simulink model "IEEE123bus_v2019b_Phasor_PI"  (R2019b)
settings: Solver=ode4  StartTime=0.0  StopTime=100  FixedStep=Ts  MaxStep=1e-4  RelTol=1e-3
InitFcn:
  | a=1; % Loading Factor
  | Ts=0.1;% For Delay Blocks in Voltage Regulator Controls
  | % phase to sequence conversion of RXB matrices
  | c=1*exp(sqrt(-1)*(120*pi/180));
  | T=[1 1 1;1 c*c c;1 c c*c];
  | Tinv=1/3*[1 1 1;1 c c*c;1 c*c c];
  | 
  | % Simulation data for the IEEE 123 Node Test Feeder model
  | mi2km = 1.60934;%  miles to km conversion
  | ft2km = 0.0003048; % feet to km conversion
  | ms2F = 1*1e-6/(2*pi*60);% microsiemens to Farads conversion
  | 
  | %% Configuration 1
  | % Series Resitance and Reactance - ohm/mile
  | R_1 = [0.4576 0.1560 0.1535;0.1560 0.4666 0.1580;0.1535 0.1580 0.4615];
  | X_1 = [1.0780 0.5017 0.3849;0.5017 1.0482 0.4236;0.3849 0.4236 1.0651];
  | % charging susceptance - microsiemens/mile
  | B_1 = [5.6765 -1.8319 -0.6982;-1.8319 5.9809 -1.1645;-0.6982 -1.1645 5.3971];
  | 
  | R_1 = R_1/mi2km;
  | Rseq=Tinv*R_1*T;
  | R1_1=Rseq(2,2);R0_1=Rseq(1,1);
  | 
  | L_1 = (X_1/(2*pi*60))/mi2km;
  | Lseq=Tinv*L_1*T;
  | L1_1=Lseq(2,2);L0_1=Lseq(1,1);
  | 
  | C_1 =(B_1*ms2F)/mi2km;
  | Cseq=Tinv*C_1*T;
  | C1_1=Cseq(2,2);C0_1=Cseq(1,1);
  | %% Configuration 2 - series reactance - ohm/mile
  | R_2 = [0.4666 0.1580 0.1560;0.1580 0.4615 0.1535;0.1560 0.1535 0.4576];
  | X_2 = [1.0482 0.4236 0.5017;0.4236 1.0651 0.3849;0.5017 0.3849 1.0780];
  | % charging susceptance - microsiemens/mile
  | B_2 = [5.9809 -1.1645 -1.8319;-1.1645 5.3971 -0.6982;-1.8319 -0.6982 5.6765];
  | 
  | R_2 = R_2/mi2km;
  | Rseq=Tinv*R_2*T;
  | R1_2=Rseq(2,2);R0_2=Rseq(1,1);
  | 
  | L_2 = (X_2/(2*pi*60))/mi2km;
  | Lseq=Tinv*L_2*T;
  | L1_2=Lseq(2,2);L0_2=Lseq(1,1);
  | 
  | C_2 =(B_2*ms2F)/mi2km;
  | Cseq=Tinv*C_2*T;
  | C1_2=Cseq(2,2);C0_2=Cseq(1,1);
  | %% Configuration 3 - series reactance - ohm/mile
  | R_3 = [0.4615 0.1535 0.1580;0.1535 0.4576 0.1560;0.1580 0.1560 0.4666];
  | X_3 = [1.0651 0.3849 0.4236;0.3849 1.0780 0.5017;0.4236 0.5017 1.0482];
  | % charging susceptance - microsiemens/mile
  | B_3 = [5.3971 -0.6982 -1.1645;-0.6982 5.6765 -1.8319; -1.1645 -1.8319 5.9809];
  | 
  | R_3 = R_3/mi2km;
  | Rseq=Tinv*R_3*T;
  | R1_3=Rseq(2,2);R0_3=Rseq(1,1);
  | 
  | L_3 = (X_3/(2*pi*60))/mi2km;
  | Lseq=Tinv*L_3*T;
  | L1_3=Lseq(2,2);L0_3=Lseq(1,1);
  | ... (+157 lines)
undefined symbols (not defined in the file or in its folder): D1, Delta, find_system, j
libraries: powerlib x771, powerlib_meascontrol x31
(part 3 of 7)

== system IEEE123bus_v2019b_Phasor_PI/38 ==
  2 : powerlib/Measurements/Three-Phase V-I Measurement  VoltageMeasurement=phase-to-ground  SetLabelV=on  LabelV=V38  Vpu=off  VpuLL=off  CurrentMeasurement=no  SetLabelI=on  LabelI=I800  Ipu=off  Pbase=100e6  Vbase=24900  OutputType=Complex  PhasorSimulation=on  PSBequivalent=0
      settings: SourceProductName=Simscape Electrical
  Ground82 : powerlib/Elements/Ground  LConnTagsString=a
      settings: SourceProductName=Simscape Electrical
  Ground83 : powerlib/Elements/Ground  LConnTagsString=a
      settings: SourceProductName=Simscape Electrical
  b : PMIOPort  Side=Right
  B : PMIOPort  Port=2  Side=Left
  connections:
  Ground82/LConn1 -- 2/RConn3 -- 2/RConn1
  Ground83/LConn1 -- 2/LConn3 -- 2/LConn1
  2/RConn2 -- b/RConn1
  2/LConn2 -- B/RConn1

== system IEEE123bus_v2019b_Phasor_PI/39 ==
  2 : powerlib/Measurements/Three-Phase V-I Measurement  VoltageMeasurement=phase-to-ground  SetLabelV=on  LabelV=V39  Vpu=off  VpuLL=off  CurrentMeasurement=no  SetLabelI=on  LabelI=I800  Ipu=off  Pbase=100e6  Vbase=24900  OutputType=Complex  PhasorSimulation=on  PSBequivalent=0
      settings: SourceProductName=Simscape Electrical
  Ground82 : powerlib/Elements/Ground  LConnTagsString=a
      settings: SourceProductName=Simscape Electrical
  Ground83 : powerlib/Elements/Ground  LConnTagsString=a
      settings: SourceProductName=Simscape Electrical
  b : PMIOPort  Side=Right
  B : PMIOPort  Port=2  Side=Left
  connections:
  2/LConn2 -- B/RConn1
  2/RConn2 -- b/RConn1
  2/LConn1 -- 2/LConn3 -- Ground83/LConn1
  2/RConn1 -- 2/RConn3 -- Ground82/LConn1

== system IEEE123bus_v2019b_Phasor_PI/4 ==
  2 : powerlib/Measurements/Three-Phase V-I Measurement  VoltageMeasurement=phase-to-ground  SetLabelV=on  LabelV=V4  Vpu=off  VpuLL=off  CurrentMeasurement=no  SetLabelI=on  LabelI=I4  Ipu=off  Pbase=100e6  Vbase=24900  OutputType=Complex  PhasorSimulation=on  PSBequivalent=0
      settings: SourceProductName=Simscape Electrical
  Ground82 : powerlib/Elements/Ground  LConnTagsString=a
      settings: SourceProductName=Simscape Electrical
  Ground83 : powerlib/Elements/Ground  LConnTagsString=a
      settings: SourceProductName=Simscape Electrical
  c : PMIOPort  Side=Right
  C : PMIOPort  Port=2  Side=Left
  connections:
  Ground83/LConn1 -- 2/LConn1 -- 2/LConn2
  Ground82/LConn1 -- 2/RConn1 -- 2/RConn2
  c/RConn1 -- 2/RConn3
  C/RConn1 -- 2/LConn3

== system IEEE123bus_v2019b_Phasor_PI/41 ==
  2 : powerlib/Measurements/Three-Phase V-I Measurement  VoltageMeasurement=phase-to-ground  SetLabelV=on  LabelV=V41  Vpu=off  VpuLL=off  CurrentMeasurement=no  SetLabelI=on  LabelI=I800  Ipu=off  Pbase=100e6  Vbase=24900  OutputType=Complex  PhasorSimulation=on  PSBequivalent=0
      settings: SourceProductName=Simscape Electrical
  Ground82 : powerlib/Elements/Ground  LConnTagsString=a
      settings: SourceProductName=Simscape Electrical
  Ground83 : powerlib/Elements/Ground  LConnTagsString=a
      settings: SourceProductName=Simscape Electrical
  c : PMIOPort  Side=Right
  C : PMIOPort  Port=2  Side=Left
  connections:
  2/LConn1 -- 2/LConn2 -- Ground83/LConn1
  2/RConn1 -- 2/RConn2 -- Ground82/LConn1
  c/RConn1 -- 2/RConn3
  C/RConn1 -- 2/LConn3

== system IEEE123bus_v2019b_Phasor_PI/43 ==
  2 : powerlib/Measurements/Three-Phase V-I Measurement  VoltageMeasurement=phase-to-ground  SetLabelV=on  LabelV=V43  Vpu=off  VpuLL=off  CurrentMeasurement=no  SetLabelI=on  LabelI=I800  Ipu=off  Pbase=100e6  Vbase=24900  OutputType=Complex  PhasorSimulation=on  PSBequivalent=0
      settings: SourceProductName=Simscape Electrical
  Ground82 : powerlib/Elements/Ground  LConnTagsString=a
      settings: SourceProductName=Simscape Electrical
  Ground83 : powerlib/Elements/Ground  LConnTagsString=a
      settings: SourceProductName=Simscape Electrical
  b : PMIOPort  Side=Right
  B : PMIOPort  Port=2  Side=Left
  connections:
  2/LConn2 -- B/RConn1
  2/RConn2 -- b/RConn1
  2/LConn1 -- 2/LConn3 -- Ground83/LConn1
  2/RConn1 -- 2/RConn3 -- Ground82/LConn1

== system IEEE123bus_v2019b_Phasor_PI/45 ==
  2 : powerlib/Measurements/Three-Phase V-I Measurement  VoltageMeasurement=phase-to-ground  SetLabelV=on  LabelV=V45  Vpu=off  VpuLL=off  CurrentMeasurement=no  SetLabelI=on  LabelI=I800  Ipu=off  Pbase=100e6  Vbase=24900  OutputType=Complex  PhasorSimulation=on  PSBequivalent=0
      settings: SourceProductName=Simscape Electrical
  Ground82 : powerlib/Elements/Ground  LConnTagsString=a
      settings: SourceProductName=Simscape Electrical
  Ground83 : powerlib/Elements/Ground  LConnTagsString=a
      settings: SourceProductName=Simscape Electrical
  a : PMIOPort  Side=Right
  A : PMIOPort  Port=2  Side=Left
  connections:
  2/RConn3 -- 2/RConn2 -- Ground82/LConn1
  2/LConn3 -- 2/LConn2 -- Ground83/LConn1
  a/RConn1 -- 2/RConn1
  A/RConn1 -- 2/LConn1

== system IEEE123bus_v2019b_Phasor_PI/46 ==
  2 : powerlib/Measurements/Three-Phase V-I Measurement  VoltageMeasurement=phase-to-ground  SetLabelV=on  LabelV=V46  Vpu=off  VpuLL=off  CurrentMeasurement=no  SetLabelI=on  LabelI=I800  Ipu=off  Pbase=100e6  Vbase=24900  OutputType=Complex  PhasorSimulation=on  PSBequivalent=0
      settings: SourceProductName=Simscape Electrical
  Ground82 : powerlib/Elements/Ground  LConnTagsString=a
      settings: SourceProductName=Simscape Electrical
  Ground83 : powerlib/Elements/Ground  LConnTagsString=a
      settings: SourceProductName=Simscape Electrical
  a : PMIOPort  Side=Right
  A : PMIOPort  Port=2  Side=Left
  connections:
  A/RConn1 -- 2/LConn1
  a/RConn1 -- 2/RConn1
  Ground83/LConn1 -- 2/LConn2 -- 2/LConn3
  Ground82/LConn1 -- 2/RConn2 -- 2/RConn3

== system IEEE123bus_v2019b_Phasor_PI/5 ==
  2 : powerlib/Measurements/Three-Phase V-I Measurement  VoltageMeasurement=phase-to-ground  SetLabelV=on  LabelV=V5  Vpu=off  VpuLL=off  CurrentMeasurement=no  SetLabelI=on  LabelI=I800  Ipu=off  Pbase=100e6  Vbase=24900  OutputType=Complex  PhasorSimulation=on  PSBequivalent=0
      settings: SourceProductName=Simscape Electrical
  Ground82 : powerlib/Elements/Ground  LConnTagsString=a
      settings: SourceProductName=Simscape Electrical
  Ground83 : powerlib/Elements/Ground  LConnTagsString=a
      settings: SourceProductName=Simscape Electrical
  c : PMIOPort  Side=Right
  C : PMIOPort  Port=2  Side=Left
  connections:
  C/RConn1 -- 2/LConn3
  c/RConn1 -- 2/RConn3
  2/RConn2 -- 2/RConn1 -- Ground82/LConn1
  2/LConn2 -- 2/LConn1 -- Ground83/LConn1

== system IEEE123bus_v2019b_Phasor_PI/58 ==
  2 : powerlib/Measurements/Three-Phase V-I Measurement  VoltageMeasurement=phase-to-ground  SetLabelV=on  LabelV=V58  Vpu=off  VpuLL=off  CurrentMeasurement=no  SetLabelI=on  LabelI=I800  Ipu=off  Pbase=100e6  Vbase=24900  OutputType=Complex  PhasorSimulation=on  PSBequivalent=0
      settings: SourceProductName=Simscape Electrical
  Ground82 : powerlib/Elements/Ground  LConnTagsString=a
      settings: SourceProductName=Simscape Electrical
  Ground83 : powerlib/Elements/Ground  LConnTagsString=a
      settings: SourceProductName=Simscape Electrical
  b : PMIOPort  Side=Right
  B : PMIOPort  Port=2  Side=Left
  connections:
  2/LConn2 -- B/RConn1
  2/RConn2 -- b/RConn1
  2/LConn1 -- 2/LConn3 -- Ground83/LConn1
  2/RConn1 -- 2/RConn3 -- Ground82/LConn1

== system IEEE123bus_v2019b_Phasor_PI/59 ==
  2 : powerlib/Measurements/Three-Phase V-I Measurement  VoltageMeasurement=phase-to-ground  SetLabelV=on  LabelV=V59  Vpu=off  VpuLL=off  CurrentMeasurement=no  SetLabelI=on  LabelI=I800  Ipu=off  Pbase=100e6  Vbase=24900  OutputType=Complex  PhasorSimulation=on  PSBequivalent=0
      settings: SourceProductName=Simscape Electrical
  Ground82 : powerlib/Elements/Ground  LConnTagsString=a
      settings: SourceProductName=Simscape Electrical
  Ground83 : powerlib/Elements/Ground  LConnTagsString=a
      settings: SourceProductName=Simscape Electrical
  b : PMIOPort  Side=Right
  B : PMIOPort  Port=2  Side=Left
  connections:
  Ground82/LConn1 -- 2/RConn3 -- 2/RConn1
  Ground83/LConn1 -- 2/LConn3 -- 2/LConn1
  2/RConn2 -- b/RConn1
  2/LConn2 -- B/RConn1

== system IEEE123bus_v2019b_Phasor_PI/6 ==
  2 : powerlib/Measurements/Three-Phase V-I Measurement  VoltageMeasurement=phase-to-ground  SetLabelV=on  LabelV=V6  Vpu=off  VpuLL=off  CurrentMeasurement=no  SetLabelI=on  LabelI=I800  Ipu=off  Pbase=100e6  Vbase=24900  OutputType=Complex  PhasorSimulation=on  PSBequivalent=0
      settings: SourceProductName=Simscape Electrical
  Ground82 : powerlib/Elements/Ground  LConnTagsString=a
      settings: SourceProductName=Simscape Electrical
  Ground83 : powerlib/Elements/Ground  LConnTagsString=a
      settings: SourceProductName=Simscape Electrical
  c : PMIOPort  Side=Right
  C : PMIOPort  Port=2  Side=Left
  connections:
  Ground83/LConn1 -- 2/LConn1 -- 2/LConn2
  Ground82/LConn1 -- 2/RConn1 -- 2/RConn2
  c/RConn1 -- 2/RConn3
  C/RConn1 -- 2/LConn3

== system IEEE123bus_v2019b_Phasor_PI/67-97 3 ==
  Config300 : powerlib/Elements/Mutual Inductance  LConnTagsString=a|b|c  RConnTagsString=A|B|C  TypeOfMutual=Generalized mutual inductance  NumberOfWindings=3  SelfImpedance1=[1.1 1.1e-03]  SelfImpedance2=[ 1.1 1.1e-03]  ThreeWindings=on  SelfImpedance3=[ 1.1 1.1e-03]  MutualImpedance=[1.0 1.0e-03]  InductanceMatrix=Ll* L  ResistanceMatrix=Rl* L  Measurements=None
      settings: AttributesFormatString=\n  SourceProductName=Simscape Electrical  SourceProductBaseCode=PS
  Ground{1..6} (6 alike) : powerlib/Elements/Ground  LConnTagsString=a
      settings: SourceProductName=Simscape Electrical
  Series RLC Branch : powerlib/Elements/Series RLC Branch  LConnTagsString=__new0  RConnTagsString=__new0  BranchType=C  Resistance=1  Inductance=1e-3  SetiL0=off  InitialCurrent=0  Capacitance=Cl(1,3)/2*L  Setx0=off  InitialVoltage=0  Measurements=None
      settings: SourceProductName=Simscape Electrical
  Series RLC Branch1 : powerlib/Elements/Series RLC Branch  LConnTagsString=__new0  RConnTagsString=__new0  BranchType=C  Resistance=1  Inductance=1e-3  SetiL0=off  InitialCurrent=0  Capacitance=Cl(1,3)/2*L  Setx0=off  InitialVoltage=0  Measurements=None
      settings: SourceProductName=Simscape Electrical
  Series RLC Branch10 : powerlib/Elements/Series RLC Branch  LConnTagsString=__new0  RConnTagsString=__new0  BranchType=C  Resistance=1  Inductance=1e-3  SetiL0=off  InitialCurrent=0  Capacitance=Cl(2,2)/2*L  Setx0=off  InitialVoltage=0  Measurements=None
      settings: SourceProductName=Simscape Electrical
  Series RLC Branch11 : powerlib/Elements/Series RLC Branch  LConnTagsString=__new0  RConnTagsString=__new0  BranchType=C  Resistance=1  Inductance=1e-3  SetiL0=off  InitialCurrent=0  Capacitance=Cl(1,1)/2*L  Setx0=off  InitialVoltage=0  Measurements=None
      settings: SourceProductName=Simscape Electrical
  Series RLC Branch2 : powerlib/Elements/Series RLC Branch  LConnTagsString=__new0  RConnTagsString=__new0  BranchType=C  Resistance=1  Inductance=1e-3  SetiL0=off  InitialCurrent=0  Capacitance=Cl(1,2)/2*L  Setx0=off  InitialVoltage=0  Measurements=None
      settings: SourceProductName=Simscape Electrical
  Series RLC Branch3 : powerlib/Elements/Series RLC Branch  LConnTagsString=__new0  RConnTagsString=__new0  BranchType=C  Resistance=1  Inductance=1e-3  SetiL0=off  InitialCurrent=0  Capacitance=Cl(2,3)/2*L  Setx0=off  InitialVoltage=0  Measurements=None
      settings: SourceProductName=Simscape Electrical
  Series RLC Branch4 : powerlib/Elements/Series RLC Branch  LConnTagsString=__new0  RConnTagsString=__new0  BranchType=C  Resistance=1  Inductance=1e-3  SetiL0=off  InitialCurrent=0  Capacitance=Cl(1,2)/2*L  Setx0=off  InitialVoltage=0  Measurements=None
      settings: SourceProductName=Simscape Electrical
  Series RLC Branch5 : powerlib/Elements/Series RLC Branch  LConnTagsString=__new0  RConnTagsString=__new0  BranchType=C  Resistance=1  Inductance=1e-3  SetiL0=off  InitialCurrent=0  Capacitance=Cl(2,3)/2*L  Setx0=off  InitialVoltage=0  Measurements=None
      settings: SourceProductName=Simscape Electrical
  Series RLC Branch6 : powerlib/Elements/Series RLC Branch  LConnTagsString=__new0  RConnTagsString=__new0  BranchType=C  Resistance=1  Inductance=1e-3  SetiL0=off  InitialCurrent=0  Capacitance=Cl(1,1)/2*L  Setx0=off  InitialVoltage=0  Measurements=None
      settings: SourceProductName=Simscape Electrical
  Series RLC Branch7 : powerlib/Elements/Series RLC Branch  LConnTagsString=__new0  RConnTagsString=__new0  BranchType=C  Resistance=1  Inductance=1e-3  SetiL0=off  InitialCurrent=0  Capacitance=Cl(2,2)/2*L  Setx0=off  InitialVoltage=0  Measurements=None
      settings: SourceProductName=Simscape Electrical
  Series RLC Branch8 : powerlib/Elements/Series RLC Branch  LConnTagsString=__new0  RConnTagsString=__new0  BranchType=C  Resistance=1  Inductance=1e-3  SetiL0=off  InitialCurrent=0  Capacitance=Cl(3,3)/2*L  Setx0=off  InitialVoltage=0  Measurements=None
      settings: SourceProductName=Simscape Electrical
  Series RLC Branch9 : powerlib/Elements/Series RLC Branch  LConnTagsString=__new0  RConnTagsString=__new0  BranchType=C  Resistance=1  Inductance=1e-3  SetiL0=off  InitialCurrent=0  Capacitance=Cl(3,3)/2*L  Setx0=off  InitialVoltage=0  Measurements=None
      settings: SourceProductName=Simscape Electrical
  A In : PMIOPort  Side=Left
  B In : PMIOPort  Port=2  Side=Left
  C in : PMIOPort  Port=3  Side=Left
  A Out : PMIOPort  Port=4  Side=Right
  B Out : PMIOPort  Port=5  Side=Right
  C Out : PMIOPort  Port=6  Side=Right
  connections:
  Series RLC Branch4/RConn1 -- Series RLC Branch5/LConn1 -- Series RLC Branch10/LConn1 -- Config300/LConn2 -- B In/RConn1
  Config300/RConn2 -- Series RLC Branch7/LConn1 -- Series RLC Branch3/LConn1 -- Series RLC Branch2/RConn1 -- B Out/RConn1
  Config300/LConn1 -- Series RLC Branch11/LConn1 -- Series RLC Branch4/LConn1 -- Series RLC Branch/LConn1 -- A In/RConn1
  Config300/RConn1 -- Series RLC Branch6/LConn1 -- Series RLC Branch2/LConn1 -- Series RLC Branch1/LConn1 -- A Out/RConn1
  Config300/LConn3 -- Series RLC Branch9/LConn1 -- Series RLC Branch5/RConn1 -- Series RLC Branch/RConn1 -- C in/RConn1
  Config300/RConn3 -- Series RLC Branch8/LConn1 -- Series RLC Branch3/RConn1 -- Series RLC Branch1/RConn1 -- C Out/RConn1
  Ground3/LConn1 -- Series RLC Branch11/RConn1
  Ground1/LConn1 -- Series RLC Branch10/RConn1
  Ground6/LConn1 -- Series RLC Branch9/RConn1
  Series RLC Branch8/RConn1 -- Ground5/LConn1
  Series RLC Branch7/RConn1 -- Ground4/LConn1
  Series RLC Branch6/RConn1 -- Ground2/LConn1

== system IEEE123bus_v2019b_Phasor_PI/68 ==
  2 : powerlib/Measurements/Three-Phase V-I Measurement  VoltageMeasurement=phase-to-ground  SetLabelV=on  LabelV=V68  Vpu=off  VpuLL=off  CurrentMeasurement=no  SetLabelI=on  LabelI=I800  Ipu=off  Pbase=100e6  Vbase=24900  OutputType=Complex  PhasorSimulation=on  PSBequivalent=0
      settings: SourceProductName=Simscape Electrical
  Ground82 : powerlib/Elements/Ground  LConnTagsString=a
      settings: SourceProductName=Simscape Electrical
  Ground83 : powerlib/Elements/Ground  LConnTagsString=a
      settings: SourceProductName=Simscape Electrical
  a : PMIOPort  Side=Right
  A : PMIOPort  Port=2  Side=Left
  connections:
  A/RConn1 -- 2/LConn1
  a/RConn1 -- 2/RConn1
  Ground83/LConn1 -- 2/LConn2 -- 2/LConn3
  Ground82/LConn1 -- 2/RConn2 -- 2/RConn3

== system IEEE123bus_v2019b_Phasor_PI/69 ==
  2 : powerlib/Measurements/Three-Phase V-I Measurement  VoltageMeasurement=phase-to-ground  SetLabelV=on  LabelV=V69  Vpu=off  VpuLL=off  CurrentMeasurement=no  SetLabelI=on  LabelI=I800  Ipu=off  Pbase=100e6  Vbase=24900  OutputType=Complex  PhasorSimulation=on  PSBequivalent=0
      settings: SourceProductName=Simscape Electrical
  Ground82 : powerlib/Elements/Ground  LConnTagsString=a
      settings: SourceProductName=Simscape Electrical
  Ground83 : powerlib/Elements/Ground  LConnTagsString=a
      settings: SourceProductName=Simscape Electrical
  a : PMIOPort  Side=Right
  A : PMIOPort  Port=2  Side=Left
  connections:
  2/RConn3 -- 2/RConn2 -- Ground82/LConn1
  2/LConn3 -- 2/LConn2 -- Ground83/LConn1
  a/RConn1 -- 2/RConn1
  A/RConn1 -- 2/LConn1

== system IEEE123bus_v2019b_Phasor_PI/70 ==
  2 : powerlib/Measurements/Three-Phase V-I Measurement  VoltageMeasurement=phase-to-ground  SetLabelV=on  LabelV=V70  Vpu=off  VpuLL=off  CurrentMeasurement=no  SetLabelI=on  LabelI=I800  Ipu=off  Pbase=100e6  Vbase=24900  OutputType=Complex  PhasorSimulation=on  PSBequivalent=0
      settings: SourceProductName=Simscape Electrical
  Ground82 : powerlib/Elements/Ground  LConnTagsString=a
      settings: SourceProductName=Simscape Electrical
  Ground83 : powerlib/Elements/Ground  LConnTagsString=a
      settings: SourceProductName=Simscape Electrical
  a : PMIOPort  Side=Right
  A : PMIOPort  Port=2  Side=Left
  connections:
  A/RConn1 -- 2/LConn1
  a/RConn1 -- 2/RConn1
  Ground83/LConn1 -- 2/LConn2 -- 2/LConn3
  Ground82/LConn1 -- 2/RConn2 -- 2/RConn3

== system IEEE123bus_v2019b_Phasor_PI/71 ==
  2 : powerlib/Measurements/Three-Phase V-I Measurement  VoltageMeasurement=phase-to-ground  SetLabelV=on  LabelV=V71  Vpu=off  VpuLL=off  CurrentMeasurement=no  SetLabelI=on  LabelI=I800  Ipu=off  Pbase=100e6  Vbase=24900  OutputType=Complex  PhasorSimulation=on  PSBequivalent=0
      settings: SourceProductName=Simscape Electrical
  Ground82 : powerlib/Elements/Ground  LConnTagsString=a
      settings: SourceProductName=Simscape Electrical
  Ground83 : powerlib/Elements/Ground  LConnTagsString=a
      settings: SourceProductName=Simscape Electrical
  a : PMIOPort  Side=Right
  A : PMIOPort  Port=2  Side=Left
  connections:
  2/RConn3 -- 2/RConn2 -- Ground82/LConn1
  2/LConn3 -- 2/LConn2 -- Ground83/LConn1
  a/RConn1 -- 2/RConn1
  A/RConn1 -- 2/LConn1

== system IEEE123bus_v2019b_Phasor_PI/73 ==
  2 : powerlib/Measurements/Three-Phase V-I Measurement  VoltageMeasurement=phase-to-ground  SetLabelV=on  LabelV=V73  Vpu=off  VpuLL=off  CurrentMeasurement=no  SetLabelI=on  LabelI=I800  Ipu=off  Pbase=100e6  Vbase=24900  OutputType=Complex  PhasorSimulation=on  PSBequivalent=0
      settings: SourceProductName=Simscape Electrical
  Ground82 : powerlib/Elements/Ground  LConnTagsString=a
      settings: SourceProductName=Simscape Electrical
  Ground83 : powerlib/Elements/Ground  LConnTagsString=a
      settings: SourceProductName=Simscape Electrical
  c : PMIOPort  Side=Right
  C : PMIOPort  Port=2  Side=Left
  connections:
  2/LConn1 -- 2/LConn2 -- Ground83/LConn1
  2/RConn1 -- 2/RConn2 -- Ground82/LConn1
  c/RConn1 -- 2/RConn3
  C/RConn1 -- 2/LConn3

== system IEEE123bus_v2019b_Phasor_PI/74 ==
  2 : powerlib/Measurements/Three-Phase V-I Measurement  VoltageMeasurement=phase-to-ground  SetLabelV=on  LabelV=V74  Vpu=off  VpuLL=off  CurrentMeasurement=no  SetLabelI=on  LabelI=I800  Ipu=off  Pbase=100e6  Vbase=24900  OutputType=Complex  PhasorSimulation=on  PSBequivalent=0
      settings: SourceProductName=Simscape Electrical
  Ground82 : powerlib/Elements/Ground  LConnTagsString=a
      settings: SourceProductName=Simscape Electrical
  Ground83 : powerlib/Elements/Ground  LConnTagsString=a
      settings: SourceProductName=Simscape Electrical
  c : PMIOPort  Side=Right
  C : PMIOPort  Port=2  Side=Left
  connections:
  C/RConn1 -- 2/LConn3
  c/RConn1 -- 2/RConn3
  Ground82/LConn1 -- 2/RConn2 -- 2/RConn1
  Ground83/LConn1 -- 2/LConn2 -- 2/LConn1

== system IEEE123bus_v2019b_Phasor_PI/75 ==
  2 : powerlib/Measurements/Three-Phase V-I Measurement  VoltageMeasurement=phase-to-ground  SetLabelV=on  LabelV=V75  Vpu=off  VpuLL=off  CurrentMeasurement=no  SetLabelI=on  LabelI=I800  Ipu=off  Pbase=100e6  Vbase=24900  OutputType=Complex  PhasorSimulation=on  PSBequivalent=0
      settings: SourceProductName=Simscape Electrical
  Ground82 : powerlib/Elements/Ground  LConnTagsString=a
      settings: SourceProductName=Simscape Electrical
  Ground83 : powerlib/Elements/Ground  LConnTagsString=a
      settings: SourceProductName=Simscape Electrical
  c : PMIOPort  Side=Right
  C : PMIOPort  Port=2  Side=Left
  connections:
  2/LConn1 -- 2/LConn2 -- Ground83/LConn1
  2/RConn1 -- 2/RConn2 -- Ground82/LConn1
  c/RConn1 -- 2/RConn3
  C/RConn1 -- 2/LConn3

== system IEEE123bus_v2019b_Phasor_PI/84 ==
  2 : powerlib/Measurements/Three-Phase V-I Measurement  VoltageMeasurement=phase-to-ground  SetLabelV=on  LabelV=V84  Vpu=off  VpuLL=off  CurrentMeasurement=no  SetLabelI=on  LabelI=I800  Ipu=off  Pbase=100e6  Vbase=24900  OutputType=Complex  PhasorSimulation=on  PSBequivalent=0
      settings: SourceProductName=Simscape Electrical
  Ground82 : powerlib/Elements/Ground  LConnTagsString=a
      settings: SourceProductName=Simscape Electrical
  Ground83 : powerlib/Elements/Ground  LConnTagsString=a
      settings: SourceProductName=Simscape Electrical
  c : PMIOPort  Side=Right
  C : PMIOPort  Port=2  Side=Left
  connections:
  C/RConn1 -- 2/LConn3
  c/RConn1 -- 2/RConn3
  Ground82/LConn1 -- 2/RConn2 -- 2/RConn1
  Ground83/LConn1 -- 2/LConn2 -- 2/LConn1

== system IEEE123bus_v2019b_Phasor_PI/85 ==
  2 : powerlib/Measurements/Three-Phase V-I Measurement  VoltageMeasurement=phase-to-ground  SetLabelV=on  LabelV=V85  Vpu=off  VpuLL=off  CurrentMeasurement=no  SetLabelI=on  LabelI=I800  Ipu=off  Pbase=100e6  Vbase=24900  OutputType=Complex  PhasorSimulation=on  PSBequivalent=0
      settings: SourceProductName=Simscape Electrical
  Ground82 : powerlib/Elements/Ground  LConnTagsString=a
      settings: SourceProductName=Simscape Electrical
  Ground83 : powerlib/Elements/Ground  LConnTagsString=a
      settings: SourceProductName=Simscape Electrical
  c : PMIOPort  Side=Right
  C : PMIOPort  Port=2  Side=Left
  connections:
  2/LConn1 -- 2/LConn2 -- Ground83/LConn1
  2/RConn1 -- 2/RConn2 -- Ground82/LConn1
  c/RConn1 -- 2/RConn3
  C/RConn1 -- 2/LConn3

== system IEEE123bus_v2019b_Phasor_PI/88 ==
  2 : powerlib/Measurements/Three-Phase V-I Measurement  VoltageMeasurement=phase-to-ground  SetLabelV=on  LabelV=V88  Vpu=off  VpuLL=off  CurrentMeasurement=no  SetLabelI=on  LabelI=I800  Ipu=off  Pbase=100e6  Vbase=24900  OutputType=Complex  PhasorSimulation=on  PSBequivalent=0
      settings: SourceProductName=Simscape Electrical
  Ground82 : powerlib/Elements/Ground  LConnTagsString=a
      settings: SourceProductName=Simscape Electrical
  Ground83 : powerlib/Elements/Ground  LConnTagsString=a
      settings: SourceProductName=Simscape Electrical
  a : PMIOPort  Side=Right
  A : PMIOPort  Port=2  Side=Left
  connections:
  A/RConn1 -- 2/LConn1
  a/RConn1 -- 2/RConn1
  2/LConn2 -- 2/LConn3 -- Ground83/LConn1
  2/RConn2 -- 2/RConn3 -- Ground82/LConn1

== system IEEE123bus_v2019b_Phasor_PI/9 ==
  2 : powerlib/Measurements/Three-Phase V-I Measurement  VoltageMeasurement=phase-to-ground  SetLabelV=on  LabelV=V9  Vpu=off  VpuLL=off  CurrentMeasurement=no  SetLabelI=on  LabelI=I800  Ipu=off  Pbase=100e6  Vbase=24900  OutputType=Complex  PhasorSimulation=on  PSBequivalent=0
      settings: SourceProductName=Simscape Electrical
  Ground82 : powerlib/Elements/Ground  LConnTagsString=a
      settings: SourceProductName=Simscape Electrical
  Ground83 : powerlib/Elements/Ground  LConnTagsString=a
      settings: SourceProductName=Simscape Electrical
  a : PMIOPort  Side=Right
  A : PMIOPort  Port=2  Side=Left
  connections:
  A/RConn1 -- 2/LConn1
  a/RConn1 -- 2/RConn1
  2/LConn2 -- 2/LConn3 -- Ground83/LConn1
  2/RConn2 -- 2/RConn3 -- Ground82/LConn1

== system IEEE123bus_v2019b_Phasor_PI/90 ==
  2 : powerlib/Measurements/Three-Phase V-I Measurement  VoltageMeasurement=phase-to-ground  SetLabelV=on  LabelV=V90  Vpu=off  VpuLL=off  CurrentMeasurement=no  SetLabelI=on  LabelI=I800  Ipu=off  Pbase=100e6  Vbase=24900  OutputType=Complex  PhasorSimulation=on  PSBequivalent=0
      settings: SourceProductName=Simscape Electrical
  Ground82 : powerlib/Elements/Ground  LConnTagsString=a
      settings: SourceProductName=Simscape Electrical
  Ground83 : powerlib/Elements/Ground  LConnTagsString=a
      settings: SourceProductName=Simscape Electrical
  b : PMIOPort  Side=Right
  B : PMIOPort  Port=2  Side=Left
  connections:
  Ground82/LConn1 -- 2/RConn3 -- 2/RConn1
  Ground83/LConn1 -- 2/LConn3 -- 2/LConn1
  2/RConn2 -- b/RConn1
  2/LConn2 -- B/RConn1

== system IEEE123bus_v2019b_Phasor_PI/92 ==
  2 : powerlib/Measurements/Three-Phase V-I Measurement  VoltageMeasurement=phase-to-ground  SetLabelV=on  LabelV=V92  Vpu=off  VpuLL=off  CurrentMeasurement=no  SetLabelI=on  LabelI=I800  Ipu=off  Pbase=100e6  Vbase=24900  OutputType=Complex  PhasorSimulation=on  PSBequivalent=0
      settings: SourceProductName=Simscape Electrical
  Ground82 : powerlib/Elements/Ground  LConnTagsString=a
      settings: SourceProductName=Simscape Electrical
  Ground83 : powerlib/Elements/Ground  LConnTagsString=a
      settings: SourceProductName=Simscape Electrical
  c : PMIOPort  Side=Right
  C : PMIOPort  Port=2  Side=Left
  connections:
  C/RConn1 -- 2/LConn3
  c/RConn1 -- 2/RConn3
  2/RConn2 -- 2/RConn1 -- Ground82/LConn1
  2/LConn2 -- 2/LConn1 -- Ground83/LConn1

== system IEEE123bus_v2019b_Phasor_PI/94 ==
  2 : powerlib/Measurements/Three-Phase V-I Measurement  VoltageMeasurement=phase-to-ground  SetLabelV=on  LabelV=V94  Vpu=off  VpuLL=off  CurrentMeasurement=no  SetLabelI=on  LabelI=I800  Ipu=off  Pbase=100e6  Vbase=24900  OutputType=Complex  PhasorSimulation=on  PSBequivalent=0
      settings: SourceProductName=Simscape Electrical
  Ground82 : powerlib/Elements/Ground  LConnTagsString=a
      settings: SourceProductName=Simscape Electrical
  Ground83 : powerlib/Elements/Ground  LConnTagsString=a
      settings: SourceProductName=Simscape Electrical
  a : PMIOPort  Side=Right
  A : PMIOPort  Port=2  Side=Left
  connections:
  Ground82/LConn1 -- 2/RConn3 -- 2/RConn2
  Ground83/LConn1 -- 2/LConn3 -- 2/LConn2
  a/RConn1 -- 2/RConn1
  A/RConn1 -- 2/LConn1

== system IEEE123bus_v2019b_Phasor_PI/96 ==
  2 : powerlib/Measurements/Three-Phase V-I Measurement  VoltageMeasurement=phase-to-ground  SetLabelV=on  LabelV=V96  Vpu=off  VpuLL=off  CurrentMeasurement=no  SetLabelI=on  LabelI=I800  Ipu=off  Pbase=100e6  Vbase=24900  OutputType=Complex  PhasorSimulation=on  PSBequivalent=0
      settings: SourceProductName=Simscape Electrical
  Ground82 : powerlib/Elements/Ground  LConnTagsString=a
      settings: SourceProductName=Simscape Electrical
  Ground83 : powerlib/Elements/Ground  LConnTagsString=a
      settings: SourceProductName=Simscape Electrical
  b : PMIOPort  Side=Right
  B : PMIOPort  Port=2  Side=Left
  connections:
  2/LConn2 -- B/RConn1
  2/RConn2 -- b/RConn1
  2/LConn1 -- 2/LConn3 -- Ground83/LConn1
  2/RConn1 -- 2/RConn3 -- Ground82/LConn1

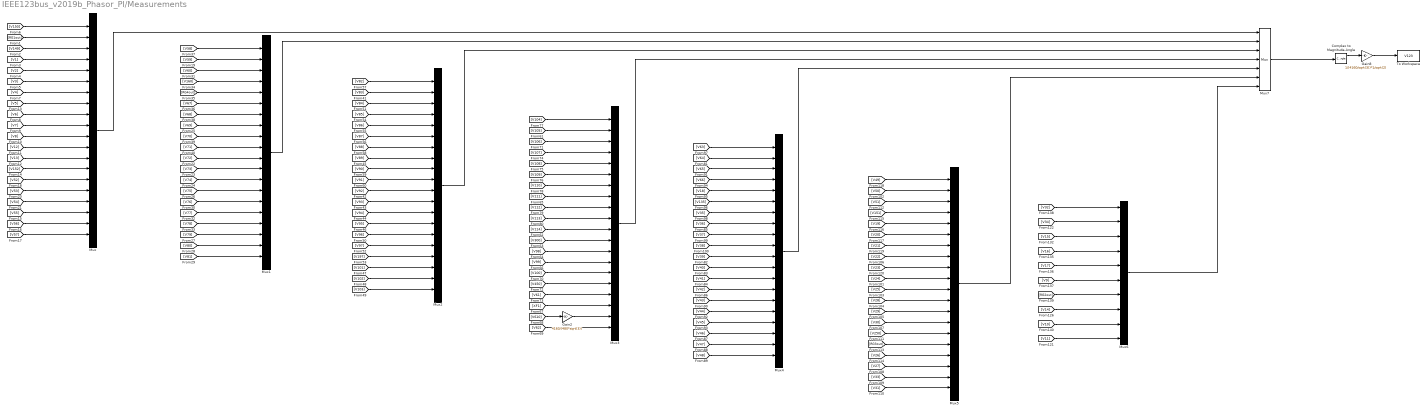
== system IEEE123bus_v2019b_Phasor_PI/Measurements ==
  Complex to Magnitude-Angle : ComplexToMagnitudeAngle
  Gain2 : Gain  Gain=4160/(480*sqrt(3))
  Gain8 : Gain  Gain=1/(4160/sqrt(3))*1/sqrt(2)
  Mux{,1..5} (6 alike) : Mux  Inputs=20
  Mux6 : Mux  Inputs=10
  Mux7 : Mux  Inputs=7
  To Workspace : ToWorkspace  VariableName=V123  SampleTime=.1
  wires:
  Gain8/1 -> To Workspace/1
  [V150] -> Mux/1
  [RG1out] -> Mux/2
  [V149] -> Mux/3
  [V1] -> Mux/4
  [V2] -> Mux/5
  [V3] -> Mux/6
  [V4] -> Mux/7
  [V5] -> Mux/8
  [V6] -> Mux/9
  [V7] -> Mux/10
  [V8] -> Mux/11
  [V12] -> Mux/12
  [V13] -> Mux/13
  [V152] -> Mux/14
  [V52] -> Mux/15
  [V53] -> Mux/16
  [V54] -> Mux/17
  [V55] -> Mux/18
  [V56] -> Mux/19
  [V57] -> Mux/20
  [V58] -> Mux1/1
  [V59] -> Mux1/2
  [V60] -> Mux1/3
  [V160] -> Mux1/4
  [RG4out] -> Mux1/5
  [V67] -> Mux1/6
  [V68] -> Mux1/7
  [V69] -> Mux1/8
  [V70] -> Mux1/9
  [V71] -> Mux1/10
  [V72] -> Mux1/11
  [V73] -> Mux1/12
  [V74] -> Mux1/13
  [V75] -> Mux1/14
  [V76] -> Mux1/15
  [V77] -> Mux1/16
  [V78] -> Mux1/17
  [V79] -> Mux1/18
  [V80] -> Mux1/19
  [V81] -> Mux1/20
  [V82] -> Mux2/1
  [V83] -> Mux2/2
  [V84] -> Mux2/3
  [V85] -> Mux2/4
  [V86] -> Mux2/5
  [V87] -> Mux2/6
  [V88] -> Mux2/7
  [V89] -> Mux2/8
  [V90] -> Mux2/9
  [V91] -> Mux2/10
  [V92] -> Mux2/11
  [V93] -> Mux2/12
  [V94] -> Mux2/13
  [V95] -> Mux2/14
  [V96] -> Mux2/15
  [V97] -> Mux2/16
  [V197] -> Mux2/17
  [V101] -> Mux2/18
  [V102] -> Mux2/19
  [V103] -> Mux2/20
  [V104] -> Mux3/1
  [V105] -> Mux3/2
  [V106] -> Mux3/3
  [V107] -> Mux3/4
  [V108] -> Mux3/5
  [V109] -> Mux3/6
  [V110] -> Mux3/7
  [V111] -> Mux3/8
  [V112] -> Mux3/9
  [V113] -> Mux3/10
  [V114] -> Mux3/11
  [V300] -> Mux3/12
  [V98] -> Mux3/13
  [V99] -> Mux3/14
  [V100] -> Mux3/15
  [V450] -> Mux3/16
  [V61] -> Mux3/17
  [XF1] -> Mux3/18
  [V610] -> Gain2/1
  [V62] -> Mux3/20
  [V63] -> Mux4/1
  [V64] -> Mux4/2
  [V65] -> Mux4/3
  [V66] -> Mux4/4
  [V18] -> Mux4/5
  [V135] -> Mux4/6
  [V35] -> Mux4/7
  [V36] -> Mux4/8
  [V37] -> Mux4/9
  [V38] -> Mux4/10
  [V39] -> Mux4/11
  [V40] -> Mux4/12
  [V41] -> Mux4/13
  [V42] -> Mux4/14
  [V43] -> Mux4/15
  [V44] -> Mux4/16
  [V45] -> Mux4/17
  [V46] -> Mux4/18
  [V47] -> Mux4/19
  [V48] -> Mux4/20
  [V49] -> Mux5/1
  [V50] -> Mux5/2
  [V51] -> Mux5/3
  [V151] -> Mux5/4
  [V19] -> Mux5/5
  [V20] -> Mux5/6
  [V21] -> Mux5/7
  [V22] -> Mux5/8
  [V23] -> Mux5/9
  [V24] -> Mux5/10
  [V25] -> Mux5/11
  [V28] -> Mux5/12
  [V29] -> Mux5/13
  [V30] -> Mux5/14
  [V250] -> Mux5/15
  [RG3out] -> Mux5/16
  [V26] -> Mux5/17
  [V27] -> Mux5/18
  [V33] -> Mux5/19
  [V31] -> Mux5/20
  Mux1/1 -> Mux7/2
  Mux/1 -> Mux7/1
  Mux2/1 -> Mux7/3
  Mux3/1 -> Mux7/4
  Mux4/1 -> Mux7/5
  Mux5/1 -> Mux7/6
  Gain2/1 -> Mux3/19
  [V32] -> Mux6/1
  [V34] -> Mux6/2
  [V15] -> Mux6/3
  [V16] -> Mux6/4
  [V17] -> Mux6/5
  [V9] -> Mux6/6
  [RG2out] -> Mux6/7
  [V14] -> Mux6/8
  [V10] -> Mux6/9
  [V11] -> Mux6/10
  Mux6/1 -> Mux7/7
  Complex to Magnitude-Angle/1 -> Gain8/1
  Mux7/1 -> Complex to Magnitude-Angle/1

== system IEEE123bus_v2019b_Phasor_PI/RG2in ==
  2 : powerlib/Measurements/Three-Phase V-I Measurement  VoltageMeasurement=phase-to-ground  SetLabelV=on  LabelV=RG2in  Vpu=off  VpuLL=off  CurrentMeasurement=no  SetLabelI=on  LabelI=I800  Ipu=off  Pbase=100e6  Vbase=24900  OutputType=Complex  PhasorSimulation=on  PSBequivalent=0
      settings: SourceProductName=Simscape Electrical
  Ground82 : powerlib/Elements/Ground  LConnTagsString=a
      settings: SourceProductName=Simscape Electrical
  Ground83 : powerlib/Elements/Ground  LConnTagsString=a
      settings: SourceProductName=Simscape Electrical
  a : PMIOPort  Side=Right
  A : PMIOPort  Port=2  Side=Left
  connections:
  A/RConn1 -- 2/LConn1
  a/RConn1 -- 2/RConn1
  2/LConn2 -- 2/LConn3 -- Ground83/LConn1
  2/RConn2 -- 2/RConn3 -- Ground82/LConn1

== system IEEE123bus_v2019b_Phasor_PI/RG2out ==
  2 : powerlib/Measurements/Three-Phase V-I Measurement  VoltageMeasurement=phase-to-ground  SetLabelV=on  LabelV=RG2out  Vpu=off  VpuLL=off  CurrentMeasurement=no  SetLabelI=on  LabelI=I800  Ipu=off  Pbase=100e6  Vbase=24900  OutputType=Complex  PhasorSimulation=on  PSBequivalent=0
      settings: SourceProductName=Simscape Electrical
  Ground82 : powerlib/Elements/Ground  LConnTagsString=a
      settings: SourceProductName=Simscape Electrical
  Ground83 : powerlib/Elements/Ground  LConnTagsString=a
      settings: SourceProductName=Simscape Electrical
  a : PMIOPort  Side=Right
  A : PMIOPort  Port=2  Side=Left
  connections:
  Ground82/LConn1 -- 2/RConn3 -- 2/RConn2
  Ground83/LConn1 -- 2/LConn3 -- 2/LConn2
  a/RConn1 -- 2/RConn1
  A/RConn1 -- 2/LConn1

== system IEEE123bus_v2019b_Phasor_PI/RG3in ==
  1 : powerlib/Measurements/Three-Phase V-I Measurement  VoltageMeasurement=phase-to-ground  SetLabelV=on  LabelV=RG3in  Vpu=off  VpuLL=off  CurrentMeasurement=no  SetLabelI=on  LabelI=I800  Ipu=off  Pbase=100e6  Vbase=24900  OutputType=Complex  PhasorSimulation=on  PSBequivalent=0
      settings: SourceProductName=Simscape Electrical
  Ground1 : powerlib/Elements/Ground  LConnTagsString=a
      settings: SourceProductName=Simscape Electrical
  Ground2 : powerlib/Elements/Ground  LConnTagsString=a
      settings: SourceProductName=Simscape Electrical
  A : PMIOPort  Side=Left
  a : PMIOPort  Port=2  Side=Right
  C : PMIOPort  Port=3  Side=Left
  c : PMIOPort  Port=4  Side=Right
  connections:
  A/RConn1 -- 1/LConn1
  a/RConn1 -- 1/RConn1
  C/RConn1 -- 1/LConn3
  1/RConn2 -- Ground1/LConn1
  c/RConn1 -- 1/RConn3
  1/LConn2 -- Ground2/LConn1

== system IEEE123bus_v2019b_Phasor_PI/RG3out ==
  1 : powerlib/Measurements/Three-Phase V-I Measurement  VoltageMeasurement=phase-to-ground  SetLabelV=on  LabelV=RG3out  Vpu=off  VpuLL=off  CurrentMeasurement=no  SetLabelI=on  LabelI=I800  Ipu=off  Pbase=100e6  Vbase=24900  OutputType=Complex  PhasorSimulation=on  PSBequivalent=0
      settings: SourceProductName=Simscape Electrical
  Ground1 : powerlib/Elements/Ground  LConnTagsString=a
      settings: SourceProductName=Simscape Electrical
  Ground2 : powerlib/Elements/Ground  LConnTagsString=a
      settings: SourceProductName=Simscape Electrical
  A : PMIOPort  Side=Left
  a : PMIOPort  Port=2  Side=Right
  C : PMIOPort  Port=3  Side=Left
  c : PMIOPort  Port=4  Side=Right
  connections:
  1/LConn2 -- Ground2/LConn1
  c/RConn1 -- 1/RConn3
  1/RConn2 -- Ground1/LConn1
  C/RConn1 -- 1/LConn3
  a/RConn1 -- 1/RConn1
  A/RConn1 -- 1/LConn1

== system IEEE123bus_v2019b_Phasor_PI/Regulator 1 ==
  Single Phase SVR_A : Subsystem  LoadFcn=find_system(gcs,'FollowLinks', 'on', 'LookUnderMasks', 'all');  mask(Single-Phase OLTC){pNom=5e6/3, fNom=60, vNom=4160/sqrt(3), ctRatio=50, ptRatio=20, DeltaU=0.00625, TapMinMax=[-16 16], InitialTap=-1, TapSelectionTime=8, RegulatorOn=on, Regulator=[120/120  2/120  12], Comp=[0.4 0.4]}
      mask prompts: pNom "Nominal Power (VA)"; fNom "Nominal Frequency (Hz)"; vNom "Nominal Voltage (Vrms)"; ctRatio "Primary CT Rating (A)"; ptRatio "PT Ratio"; DeltaU "Voltage Step Per Tap (pu)"; TapMinMax "Minimum and Maximum Tap Positions"; InitialTap "Initial Tap Position"; TapSelectionTime "Tap Selection Time (s)"; RegulatorOn "Voltage Regulator"; Regulator "Voltage Regulator [ Vref(pu) DeadBand(pu)  Delay(s)]"; Comp "Compensator Settings [R (V) X(V)]"
      mask help:
      | Models a single-phase On Load Tap Changer (OLTC). The single-phase primary of multi-tap winding is modeled with a Variable-Ratio Transformer block.
      |
      | The transformer voltage ratio U2/U1 (in pu) is given by:
      |                 U2/U1= 1/ (1+TapPosition*DeltaU)
      | Tap position 0 corresponds to nominal voltage ratio.
      |
      | When Voltage regulator is 'on',  voltage regulator asks for a tap change if:
      |                  abs(Vm-Vref)>DeadBand/2  during a time  t > Delay.
      |
      | where 'Vm' is voltage measured at regulating point and Vref is reference voltage.
      | With line drop compensation, Vm=Vsec-Isec(R+jX)
      mask init:
      | RegulatorVref=Regulator(1);
      | RegulatorDeadBand=Regulator(2);
      | RegulatorDelay=Regulator(3);
      | Rc=Comp(1);
      | Xc=Comp(2);
      mask TypeOptions RegulatorOn: off | on
      mask Callback RegulatorOn:
      | tempMaskVis=get_param(gcb,'MaskVisibilities');
      | if strcmp(get_param(gcb,'RegulatorOn'),'on')
      | 	tempMaskVis{11}='on';
      | 	set_param(gcb,'MaskVisibilities',tempMaskVis);
      | else
      | 	tempMaskVis{11}='off';
      | 	set_param(gcb,'MaskVisibilities',tempMaskVis);
      | end
      | if strcmp(get_param(gcb,'RegulatorOn'),'on')
      | 	tempMaskVis{12}='on';
      | 	set_param(gcb,'MaskVisibilities',tempMaskVis);
      | else
      | 	tempMaskVis{12}='off';
      | 	set_param(gcb,'MaskVisibilities',tempMaskVis);
      | end
      mask DialogControl Container8 Prompt: Setup
      mask DialogControl Container13 Prompt: Regulator Parameters
  A : PMIOPort  Side=Left
  a : PMIOPort  Port=2  Side=Right
  Tap : Outport
  wires:
  Single Phase SVR_A/1(Tap) -> Tap/1
  connections:
  Single Phase SVR_A/RConn1 -- a/RConn1
  Single Phase SVR_A/LConn1 -- A/RConn1

== system IEEE123bus_v2019b_Phasor_PI/Regulator 1 Three Phase Ganged SVR ==
  note: Here the voltage of one phase is used to control taps of all phases
      | The phase A voltage is monitored and used to control taps of other phases
  Ganged Line Drop Compensator : Subsystem  mask{pNom=5e6/3, fNom=60, vNom=4160/sqrt(3), ptRatio=20, Comp=[3 7.5]}
      mask prompts: pNom "Nominal power (VA)"; fNom "Nominal frequency (Hz)"; vNom "Nominal voltage (Vrms)"; ptRatio "PT Ratio"; Comp "Compensator Settings [R (V) X(V)]"
      mask init:
      | Rc=Comp(1);
      | Xc=Comp(2);
  Mux : Mux  Inputs=3
  Single Phase SVR_A : Subsystem  LoadFcn=find_system(gcs,'FollowLinks', 'on', 'LookUnderMasks', 'all');  mask(Single-Phase OLTC){pNom=5e6/3, fNom=60, vNom=4160/sqrt(3), ctRatio=700, ptRatio=20, DeltaU=0.00625, TapMinMax=[-16 16], InitialTap=7, TapSelectionTime=8, RegulatorOn=on, Regulator=[120/120  2/120  2]}
      mask prompts: pNom "Nominal Power (VA)"; fNom "Nominal Frequency (Hz)"; vNom "Nominal Voltage (Vrms)"; ctRatio "Primary CT Rating (A)"; ptRatio "PT Ratio"; DeltaU "Voltage Step Per Tap (pu)"; TapMinMax "Minimum and Maximum Tap Positions"; InitialTap "Initial Tap Position"; TapSelectionTime "Tap Selection Time (s)"; RegulatorOn "Voltage Regulator"; Regulator "Voltage Regulator [ Vref(pu) DeadBand(pu)  Delay(s)]"
      mask help:
      | Models a single-phase On Load Tap Changer (OLTC). The single-phase primary of multi-tap winding is modeled with a Variable-Ratio Transformer block.
      |
      | The transformer voltage ratio U2/U1 (in pu) is given by:
      |                 U2/U1= 1/ (1+TapPosition*DeltaU)
      | Tap position 0 corresponds to nominal voltage ratio.
      |
      | When Voltage regulator is 'on',  voltage regulator asks for a tap change if:
      |                  abs(Vm-Vref)>DeadBand/2  during a time  t > Delay.
      |
      | where 'Vm' is voltage measured at regulating point and Vref is reference voltage.
      | With line drop compensation, Vm=Vsec-Isec(R+jX)
      mask init:
      | RegulatorVref=Regulator(1);
      | RegulatorDeadBand=Regulator(2);
      | RegulatorDelay=Regulator(3);
      mask TypeOptions RegulatorOn: off | on
      mask Callback RegulatorOn:
      | tempMaskVis=get_param(gcb,'MaskVisibilities');
      | if strcmp(get_param(gcb,'RegulatorOn'),'on')
      | 	tempMaskVis{11}='on';
      | 	set_param(gcb,'MaskVisibilities',tempMaskVis);
      | else
      | 	tempMaskVis{11}='off';
      | 	set_param(gcb,'MaskVisibilities',tempMaskVis);
      | end
      mask DialogControl Container8 Prompt: Setup
      mask DialogControl Container13 Prompt: Regulator Parameters
  Single Phase SVR_B : Subsystem  LoadFcn=find_system(gcs,'FollowLinks', 'on', 'LookUnderMasks', 'all');  mask(Single-Phase OLTC){pNom=5e6/3, fNom=60, vNom=4160/sqrt(3), ctRatio=700, ptRatio=20, DeltaU=0.00625, TapMinMax=[-16 16], InitialTap=7, TapSelectionTime=8, RegulatorOn=on, Regulator=[120/120  2/120  2]}
      mask prompts: pNom "Nominal Power (VA)"; fNom "Nominal Frequency (Hz)"; vNom "Nominal Voltage (Vrms)"; ctRatio "Primary CT Rating (A)"; ptRatio "PT Ratio"; DeltaU "Voltage Step Per Tap (pu)"; TapMinMax "Minimum and Maximum Tap Positions"; InitialTap "Initial Tap Position"; TapSelectionTime "Tap Selection Time (s)"; RegulatorOn "Voltage Regulator"; Regulator "Voltage Regulator [ Vref(pu) DeadBand(pu)  Delay(s)]"
      mask help:
      | Models a single-phase On Load Tap Changer (OLTC). The single-phase primary of multi-tap winding is modeled with a Variable-Ratio Transformer block.
      |
      | The transformer voltage ratio U2/U1 (in pu) is given by:
      |                 U2/U1= 1/ (1+TapPosition*DeltaU)
      | Tap position 0 corresponds to nominal voltage ratio.
      |
      | When Voltage regulator is 'on',  voltage regulator asks for a tap change if:
      |                  abs(Vm-Vref)>DeadBand/2  during a time  t > Delay.
      |
      | where 'Vm' is voltage measured at regulating point and Vref is reference voltage.
      | With line drop compensation, Vm=Vsec-Isec(R+jX)
      mask init:
      | RegulatorVref=Regulator(1);
      | RegulatorDeadBand=Regulator(2);
      | RegulatorDelay=Regulator(3);
      mask TypeOptions RegulatorOn: off | on
      mask Callback RegulatorOn:
      | tempMaskVis=get_param(gcb,'MaskVisibilities');
      | if strcmp(get_param(gcb,'RegulatorOn'),'on')
      | 	tempMaskVis{11}='on';
      | 	set_param(gcb,'MaskVisibilities',tempMaskVis);
      | else
      | 	tempMaskVis{11}='off';
      | 	set_param(gcb,'MaskVisibilities',tempMaskVis);
      | end
      mask DialogControl Container8 Prompt: Setup
      mask DialogControl Container13 Prompt: Regulator Parameters
  Single Phase SVR_C : Subsystem  LoadFcn=find_system(gcs,'FollowLinks', 'on', 'LookUnderMasks', 'all');  mask(Single-Phase OLTC){pNom=5e6/3, fNom=60, vNom=4160/sqrt(3), ctRatio=700, ptRatio=20, DeltaU=0.00625, TapMinMax=[-16 16], InitialTap=7, TapSelectionTime=8, RegulatorOn=on, Regulator=[120/120  2/120  2]}
      mask prompts: pNom "Nominal Power (VA)"; fNom "Nominal Frequency (Hz)"; vNom "Nominal Voltage (Vrms)"; ctRatio "Primary CT Rating (A)"; ptRatio "PT Ratio"; DeltaU "Voltage Step Per Tap (pu)"; TapMinMax "Minimum and Maximum Tap Positions"; InitialTap "Initial Tap Position"; TapSelectionTime "Tap Selection Time (s)"; RegulatorOn "Voltage Regulator"; Regulator "Voltage Regulator [ Vref(pu) DeadBand(pu)  Delay(s)]"
      mask help:
      | Models a single-phase On Load Tap Changer (OLTC). The single-phase primary of multi-tap winding is modeled with a Variable-Ratio Transformer block.
      |
      | The transformer voltage ratio U2/U1 (in pu) is given by:
      |                 U2/U1= 1/ (1+TapPosition*DeltaU)
      | Tap position 0 corresponds to nominal voltage ratio.
      |
      | When Voltage regulator is 'on',  voltage regulator asks for a tap change if:
      |                  abs(Vm-Vref)>DeadBand/2  during a time  t > Delay.
      |
      | where 'Vm' is voltage measured at regulating point and Vref is reference voltage.
      | With line drop compensation, Vm=Vsec-Isec(R+jX)
      mask init:
      | RegulatorVref=Regulator(1);
      | RegulatorDeadBand=Regulator(2);
      | RegulatorDelay=Regulator(3);
      mask TypeOptions RegulatorOn: off | on
      mask Callback RegulatorOn:
      | tempMaskVis=get_param(gcb,'MaskVisibilities');
      | if strcmp(get_param(gcb,'RegulatorOn'),'on')
      | 	tempMaskVis{11}='on';
      | 	set_param(gcb,'MaskVisibilities',tempMaskVis);
      | else
      | 	tempMaskVis{11}='off';
      | 	set_param(gcb,'MaskVisibilities',tempMaskVis);
      | end
      mask DialogControl Container8 Prompt: Setup
      mask DialogControl Container13 Prompt: Regulator Parameters
  A : PMIOPort  Side=Left
  a : PMIOPort  Port=2  Side=Right
  B : PMIOPort  Port=3  Side=Left
  b : PMIOPort  Port=4  Side=Right
  C : PMIOPort  Port=5  Side=Left
  c : PMIOPort  Port=6  Side=Right
  Tap : Outport
  tag scope: Vr1=global
  wires:
  [Vm] -> Single Phase SVR_C/1(Vm)
  [Vm] -> Single Phase SVR_B/1(Vm)
  [Vm] -> Single Phase SVR_A/1(Vm)
  Ganged Line Drop Compensator/1(Vm) -> [Vr1], [Vm]
  Single Phase SVR_A/3(Vsec) -> Ganged Line Drop Compensator/2(Vsec)
  Single Phase SVR_A/2(Isec) -> Ganged Line Drop Compensator/1(Isec)
  Single Phase SVR_A/1(Tap) -> Mux/1
  Single Phase SVR_B/1(Tap) -> Mux/2
  Single Phase SVR_C/1(Tap) -> Mux/3
  Mux/1 -> Tap/1
  connections:
  Single Phase SVR_A/RConn1 -- a/RConn1
  Single Phase SVR_A/LConn1 -- A/RConn1
  Single Phase SVR_B/LConn1 -- B/RConn1
  Single Phase SVR_B/RConn1 -- b/RConn1
  Single Phase SVR_C/LConn1 -- C/RConn1
  Single Phase SVR_C/RConn1 -- c/RConn1
